simulink model "Bulk_SM_SM_SE_Sim"  (R2015a)
settings: Solver=ode4  StartTime=0.0  StopTime=tf  FixedStep=t_step  RelTol=1e-3
values from neighbouring files (symbols this model uses):
  A = [ -1/(R*Cp), 1/Cp; -1/L, 0]    [Bulk_FL_PP_SE.m]    (also in Bulk_SM_PP_SE.m; Bulk_SM_SM_SE.m)
  B = [0;  Vi/L]    [Bulk_FL_PP_SE.m]    (also in Bulk_SM_PP_SE.m; Bulk_SM_SM_SE.m)
  C = [1, 0]    [Bulk_FL_PP_SE.m]    (also in Bulk_SM_PP_SE.m; Bulk_SM_SM_SE.m)
  Cp = 50e-6    (= 5e-05)    [BulkMod_SMIA_SMIA.m]    (also in Bulk_FL_PP_SE.m; Bulk_SM_PP_SE.m; Bulk_SM_SM_SE.m)
  DB = 1 - 2*L/(Ts*R)    (= 0.8)    [BulkMod_SMIA_SMIA.m]    (also in Bulk_FL_PP_SE.m; Bulk_SM_PP_SE.m; Bulk_SM_SM_SE.m)
  DBm = DB * Ts / (2*L)    (= 0.04)    [BulkMod_SMIA_SMIA.m]    (also in Bulk_FL_PP_SE.m; Bulk_SM_PP_SE.m; Bulk_SM_SM_SE.m)
  Ks = 200 * Vi * lambda / ts    [BulkMod_SMIA_SMIA.m]    (also in Bulk_SM_PP_SE.m = 2 * Vi * (1 + lambda) / ts; Bulk_SM_SM_SE.m = Vi * (1 + lambda) / ts)
  L = 100e-6    (= 0.0001)    [BulkMod_SMIA_SMIA.m]    (also in Bulk_FL_PP_SE.m; Bulk_SM_PP_SE.m; Bulk_SM_SM_SE.m)
  L_fpe = place(A', C', P_obs)'    [Bulk_FL_PP_SE.m]    (also in Bulk_SM_PP_SE.m; Bulk_SM_SM_SE.m)
  lambda = 700    [BulkMod_SMIA_SMIA.m]    (also in Bulk_SM_PP_SE.m = 450; Bulk_SM_SM_SE.m)
  phi = 0.001 * lambda^2    [BulkMod_SMIA_SMIA.m]    (also in Bulk_SM_PP_SE.m = 0.01 * lambda; Bulk_SM_SM_SE.m = 0.001 * lambda)
  R = 100    [BulkMod_SMIA_SMIA.m]    (also in Bulk_FL_PP_SE.m; Bulk_SM_PP_SE.m; Bulk_SM_SM_SE.m)
  Ts = 1e-5    (= 1e-05)    [BulkMod_SMIA_SMIA.m]    (also in Bulk_FL_PP_SE.m; Bulk_SM_PP_SE.m; Bulk_SM_SM_SE.m)
  Vi = 30    [BulkMod_SMIA_SMIA.m]    (also in Bulk_FL_PP_SE.m; Bulk_SM_PP_SE.m; Bulk_SM_SM_SE.m)
libraries: simulink x1
settings Model: Creator=Marcelo  LastModifiedBy=Marcelo

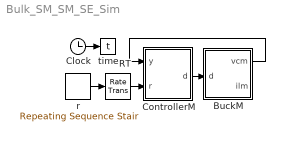
== system Bulk_SM_SM_SE_Sim ==
  BuckM : Subsystem
  Clock : Clock
  ControllerM : Subsystem
  RT : RateTransition  Integrity=off  Deterministic=off  X0=2
  r : simulink/Sources/Repeating Sequence Stair  OutValues=[2, 26, 14].'  tsamp=Tr  OutMin=[]  OutMax=[]  OutDataTypeStr=double  OutputDataTypeScalingMode=double  OutDataType=fixdt(0,8)  ConRadixGroup=Best Precision: Vector-wise  OutScaling=2^-12
  time : ToWorkspace  VariableName=t  SampleTime=-1
  wires:
  Clock/1 -> time/1
  BuckM/1(vcm) -> ControllerM/1(y)
  r/1 -> RT/1
  RT/1 -> ControllerM/2(r)
  ControllerM/1(d) -> BuckM/1(d)

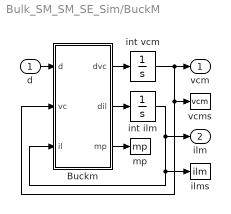
== system Bulk_SM_SM_SE_Sim/BuckM ==
  d : Inport
  Buckm : MATLAB Function  TreatAsAtomicUnit=on
  ilms : ToWorkspace  VariableName=ilm  SampleTime=-1
  int ilm : Integrator  LimitOutput=on  LowerSaturationLimit=0
  int vcm : Integrator  LimitOutput=on  LowerSaturationLimit=0
  mp : ToWorkspace  VariableName=mp  SampleTime=-1
  vcms : ToWorkspace  VariableName=vcm  SampleTime=-1
  vcm : Outport
  ilm : Outport  Port=2
  wires:
  int ilm/1 -> Buckm/3(il), ilms/1, ilm/1
  d/1 -> Buckm/1(d)
  int vcm/1 -> Buckm/2(vc), vcms/1, vcm/1
  Buckm/1(dvc) -> int vcm/1
  Buckm/2(dil) -> int ilm/1
  Buckm/3(mp) -> mp/1

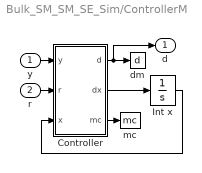
== system Bulk_SM_SM_SE_Sim/ControllerM ==
  y : Inport
  r : Inport  Port=2
  Controller : MATLAB Function  TreatAsAtomicUnit=on
  Int x : Integrator  InitialCondition=[0; 0]  LimitOutput=on  UpperSaturationLimit=[2*Vi; 2*Vi/R]  LowerSaturationLimit=[0; 0]
  dm : ToWorkspace  VariableName=d  SampleTime=-1
  mc : ToWorkspace  VariableName=mc  SampleTime=-1
  d : Outport
  wires:
  Controller/1(d) -> dm/1, d/1
  y/1 -> Controller/1(y)
  r/1 -> Controller/2(r)
  Controller/3(mc) -> mc/1
  Controller/2(dx) -> Int x/1
  Int x/1 -> Controller/3(x)

== matlab function Bulk_SM_SM_SE_Sim/BuckM/Buckm ==
  data: d input; dvc output; vc input; il input; Vi parameter; R parameter; L parameter; Cp parameter; dil output; Ts parameter; DB parameter; mp output
function [dvc, dil, mp] = fcn(d, vc, il, Vi, R, L, Cp, Ts, DB)
DBm = DB * Ts / (2*L);
ilb = DBm * (Vi - vc);
if il < ilb % Nonlinear
    dvc = il/Cp - vc/(R*Cp);
    dil = Vi*d/L - 2*il*vc/(d*Ts*(Vi-vc));
    mp = 0;
else % Linear
    dvc = il/Cp - vc/(R*Cp);
    dil = Vi*d/L - vc/L;
    mp = 1;
end

== matlab function Bulk_SM_SM_SE_Sim/ControllerM/Controller ==
  data: y input; r input; x input; R parameter; Cp parameter; L parameter; Vi parameter; Ts parameter; d output; DBm parameter; dx output; mc output size=1; lambda parameter; phi parameter; Ks parameter; A parameter; B parameter; C parameter; L_fpe parameter
function [d, dx, mc] = fcn(y, r, x, R, Cp, L, Vi, Ts, DBm, lambda, phi, Ks, A, B, C, L_fpe)
vcm = x(1);
ilm = x(2);
ilb = DBm * (Vi - vcm); % Conduction Mode Boundary
dvcm = (ilm - vcm/R) / Cp;
% Sliding Surface
s = dvcm + lambda * (vcm - r);
% Slinding-Mode Controller
sat_s = min(1, max(-1, s/phi));
v = - lambda * dvcm - Ks * sat_s;
if ilm < ilb %%%   NONLINEAR   %%%
    % Controller - Input-Output Linearization
    a = L * (ilm/(R*Cp) - vcm/(R^2*Cp) + Cp*v) / (2*Vi);
    b = 2 * ilm * vcm * L / (Vi * Ts * (Vi - vcm));
    d = a + sqrt(a^2 + b);
    % Observer - Nonlinear Luenberguer
    dx = [dvcm; Vi*d/L-2*ilm*vcm/(d*Ts*(Vi-vcm))] + L_fpe * (y - C*x);
    mc = 0;
else         %%%   LINEAR      %%%
    % Controller - Pole Placement with Tracking
    d = (L * (Cp*v + (ilm - vcm/R) / (R*Cp)) + vcm) / Vi;
    % Observer - Linear Luenberguer
    dx = A*x + B*d + L_fpe * (y - C*x);
    mc = 1;
end

if d > 1
    d = 1;
elseif d < 1e-10
    d = 1e-10;
end
